simulink model "prb_4th"  (R2020a)
settings: Solver=VariableStepAuto  StartTime=0.0  StopTime=10.0  RelTol=1e-3
settings Model: Creator=Riyansh  LastModifiedBy=Riyansh

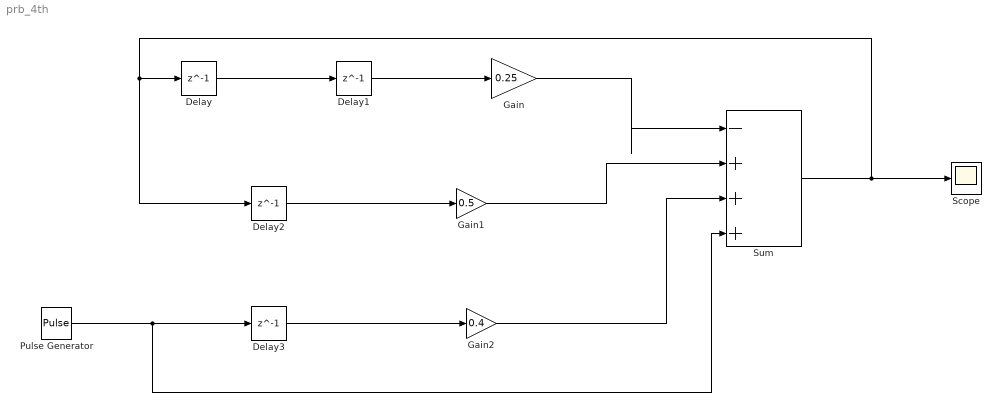
== system prb_4th ==
  Delay{,1..3} (4 alike) : Delay  DelayLength=1
  Gain : Gain  Gain=0.25
  Gain1 : Gain  Gain=0.5
  Gain2 : Gain  Gain=0.4
  Pulse Generator : DiscretePulseGenerator  PulseType=Time based  Period=10  PulseWidth=5
  Scope : Scope
  Sum : Sum  Inputs=|-+++
  wires:
  Delay2/1 -> Gain1/1
  Delay3/1 -> Gain2/1
  Delay1/1 -> Gain/1
  Delay/1 -> Delay1/1
  Gain/1 -> Sum/1
  Gain1/1 -> Sum/2
  Sum/1 -> Delay/1, Delay2/1, Scope/1
  Gain2/1 -> Sum/3
  Pulse Generator/1 -> Sum/4, Delay3/1
